simulink model "full_simulation_split_hil_new_connection"  (Simulink 7.9)
settings: Solver=ode1  StartTime=0  StopTime=10  FixedStep=Ts  RelTol=1e-8
values from neighbouring files (symbols this model uses):
  A_fx = 2e-2 * 0.4    (= 0.008)    [QR_DI_Init.m]    (also in quadro_cascade_disturbance_wo_wind.m)
  A_fy = A_fx    (= 0.008)    [QR_DI_Init.m]    (also in quadro_cascade_disturbance_wo_wind.m)
  A_fz = 2 * A_fx    (= 0.016)    [QR_DI_Init.m]    (also in quadro_cascade_disturbance_wo_wind.m)
  Bias_Phi = -0.0088    [QR_DI_Init.m]    (also in Reference_Calibration.m = mean(Phi))
  Bias_Theta = 0.022    [QR_DI_Init.m]    (also in Reference_Calibration.m = mean(Theta))
  command_on = 1    [QR_DI_Init.m]    (also in quadro_cascade_disturbance_wo_wind.m)
  cw_x = 1.05    [QR_DI_Init.m]    (also in quadro_cascade_disturbance_wo_wind.m)
  cw_y = cw_x    (= 1.05)    [QR_DI_Init.m]    (also in quadro_cascade_disturbance_wo_wind.m)
  cw_z = 1.05    [QR_DI_Init.m]    (also in quadro_cascade_disturbance_wo_wind.m)
  deltaTm = 0.2    [QR_DI_Init.m]    (also in quadro_cascade_disturbance_wo_wind.m)
  den_psi_ref = poly( ones(1,2) * -1 * T_psi_ref)    [QR_DI_Init.m]    (also in quadro_cascade_disturbance_wo_wind.m)
  den_x_ref = poly( ones(1,4) * -1 * T_x_ref)    [QR_DI_Init.m]    (also in quadro_cascade_disturbance_wo_wind.m)
  den_y_ref = poly( ones(1,4) * -1 * T_y_ref)    [QR_DI_Init.m]    (also in quadro_cascade_disturbance_wo_wind.m)
  den_z_ref = poly( ones(1,4) * -1 * T_z_ref)    [QR_DI_Init.m]    (also in quadro_cascade_disturbance_wo_wind.m)
  drot = 0.0117    [QR_DI_Init.m]    (also in quadro_cascade_disturbance_wo_wind.m = 0.2)
  dtran = 0.01    [QR_DI_Init.m]    (also in quadro_cascade_disturbance_wo_wind.m = 0.003)
  Fz_gain = 1 + 0.05*rand(1)    [QR_DI_Init.m]    (also in quadro_cascade_disturbance_wo_wind.m)
  Fz_lo = - 1.2 * m * g    (= -3.5316)    [QR_DI_Init.m]    (also in quadro_cascade_disturbance_wo_wind.m = -4.1202)
  Fz_up = 0    [QR_DI_Init.m]    (also in quadro_cascade_disturbance_wo_wind.m)
  g = 9.81    [QR_DI_Init.m]    (also in quadro_cascade_disturbance_wo_wind.m)
  Iq = [I_xx 0 0 ; 0 I_yy 0 ; 0 0 I_zz ]    [QR_DI_Init.m]    (also in quadro_cascade_disturbance_wo_wind.m = [0.0605 0 0; 0 0.0605 0; 0 0 0.018])
  K_err = old(:,2:end)    [QR_DI_Init.m]    (also in quadro_cascade_disturbance_wo_wind.m)
  K_Mot_Force = 0.3512    [QR_DI_Init.m]    (also in quadro_cascade_disturbance_wo_wind.m)
  K_Mot_Torque = 0.013    [QR_DI_Init.m]    (also in quadro_cascade_disturbance_wo_wind.m = 0.0013)
  l = 0.25    [QR_DI_Init.m]    (also in quadro_cascade_disturbance_wo_wind.m = 0.2775)
  m = 0.30    (= 0.3)    [QR_DI_Init.m]    (also in quadro_cascade_disturbance_wo_wind.m)
  m_real = m * ( 1 + 0.05*rand(1))    [QR_DI_Init.m]    (also in quadro_cascade_disturbance_wo_wind.m)
  Mm = 0.0    (= 0)    [QR_DI_Init.m]    (also in quadro_cascade_disturbance_wo_wind.m = 0.5)
  Mx_lo = - Mx_up    (= -0.2)    [QR_DI_Init.m]    (also in quadro_cascade_disturbance_wo_wind.m)
  Mx_up = 0.20    (= 0.2)    [QR_DI_Init.m]    (also in quadro_cascade_disturbance_wo_wind.m)
  My_lo = - My_up    (= -0.2)    [QR_DI_Init.m]    (also in quadro_cascade_disturbance_wo_wind.m)
  My_up = 0.20    (= 0.2)    [QR_DI_Init.m]    (also in quadro_cascade_disturbance_wo_wind.m)
  Mz_lo = - Mz_up    (= -0.02)    [QR_DI_Init.m]    (also in quadro_cascade_disturbance_wo_wind.m = -0.002)
  Mz_up = 0.02    [QR_DI_Init.m]    (also in quadro_cascade_disturbance_wo_wind.m = 0.002)
  phase_wind_z = 0    [QR_DI_Init.m]    (also in quadro_cascade_disturbance_wo_wind.m)
  psi_p_lim = 10*pi/180    (= 0.174532925199)    [QR_DI_Init.m]    (also in quadro_cascade_disturbance_wo_wind.m = 5)
  PWM_MAX = 200    [QR_DI_Init.m]    (also in quadro_cascade_disturbance_wo_wind.m)
  rho_air = 1.2041    [QR_DI_Init.m]    (also in quadro_cascade_disturbance_wo_wind.m)
  sample_time_noise_psi = 0.1    [QR_DI_Init.m]
  sample_time_noise_x = 0.2    [QR_DI_Init.m]
  sample_time_noise_y = 0.2    [QR_DI_Init.m]
  sample_time_noise_z = 0.1    [QR_DI_Init.m]
  seed_psi = seedvector(7)    [QR_DI_Init.m]
  seed_x = seedvector(1)    [QR_DI_Init.m]    (also in quadro_cascade_disturbance_wo_wind.m)
  seed_xp = seedvector(4)    [QR_DI_Init.m]    (also in quadro_cascade_disturbance_wo_wind.m)
  seed_y = seedvector(2)    [QR_DI_Init.m]    (also in quadro_cascade_disturbance_wo_wind.m)
  seed_yp = seedvector(5)    [QR_DI_Init.m]    (also in quadro_cascade_disturbance_wo_wind.m)
  seed_z = seedvector(3)    [QR_DI_Init.m]    (also in quadro_cascade_disturbance_wo_wind.m)
  seed_zp = seedvector(6)    [QR_DI_Init.m]    (also in quadro_cascade_disturbance_wo_wind.m)
  std_dev_psi = 1 * pi/180 * Noise_on    (= 0)    [QR_DI_Init.m]
  std_dev_x = 1e-1 * Noise_on    (= 0)    [QR_DI_Init.m]
  std_dev_xp = 0.03 * Noise_on    (= 0)    [QR_DI_Init.m]
  std_dev_y = 1e-1 * Noise_on    (= 0)    [QR_DI_Init.m]
  std_dev_yp = 0.03 * Noise_on    (= 0)    [QR_DI_Init.m]
  std_dev_z = 0.03 * Noise_on    (= 0)    [QR_DI_Init.m]
  std_dev_zp = 0.03 * Noise_on    (= 0)    [QR_DI_Init.m]
  T_refalt = 0.01    [QR_DI_Init.m]    (also in quadro_cascade_disturbance_wo_wind.m)
  T_wind_z = 24    [QR_DI_Init.m]    (also in quadro_cascade_disturbance_wo_wind.m)
  Tm = 10    [QR_DI_Init.m]    (also in quadro_cascade_disturbance_wo_wind.m)
  Ts = 1e-2    (= 0.01)    [QR_DI_Init.m]    (also in quadro_cascade_disturbance_wo_wind.m)
  v_wind_max_z = 2    [QR_DI_Init.m]    (also in quadro_cascade_disturbance_wo_wind.m)
  wind_on = 0    [QR_DI_Init.m]    (also in quadro_cascade_disturbance_wo_wind.m)
  x_p_lim = 1.5    [QR_DI_Init.m]    (also in quadro_cascade_disturbance_wo_wind.m = 5)
  y_p_lim = 1.5    [QR_DI_Init.m]    (also in quadro_cascade_disturbance_wo_wind.m = 5)
  z_p_lim = 1    [QR_DI_Init.m]    (also in quadro_cascade_disturbance_wo_wind.m = 1.5)
undefined symbols (not defined in the file or in its folder): T_wind_fine, v_wind_x_fine, v_wind_y_fine
libraries: simulink x5, dspsigops x4, Ports x4, aerolibtransform2 x3, dspmtrx3 x1, aerolibutil x1
(part 3 of 6)

== matlab function Error Dynamic/coordinate transformation1/Embedded MATLAB Function ==
  data: xwhole_ext input double size=[14 1]; xi output double size=14; m input double; I input double size=[3 3]; dtran input double; drot input double
% S.H. 26.03.2013
% new correct coordinate transformation

function xi  = fcn(xwhole_ext, m, I, dtran, drot)
% This block supports the Embedded MATLAB subset.
% See the help menu for details. 
x = xwhole_ext(1);
y = xwhole_ext(2);
z = xwhole_ext(3);
dx = xwhole_ext(4);
dy = xwhole_ext(5);
dz = xwhole_ext(6);

% phi = xwhole_ext(7);
% theta = xwhole_ext(8);
% psi = xwhole_ext(9);
% p = xwhole_ext(10);
% q = xwhole_ext(11);
% r = xwhole_ext(12);
% 
% xi1 = xwhole_ext(13) +eps;
% dxi1 = xwhole_ext(14) +eps;

% S.H. 26.03.2013 --> in order to match "controller_design_steps.m"
phi_angle = xwhole_ext(7);
theta_angle = xwhole_ext(8);
psi_angle = xwhole_ext(9);
p = xwhole_ext(10);
q = xwhole_ext(11);
r = xwhole_ext(12);

Sym_zeta    = xwhole_ext(13) +eps;
Sym_zeta_p  = xwhole_ext(14) +eps;


%g = -9.81;
g = 9.81;   % S.H. 26.03.2013


Ixx = I(1,1);
Ixy = I(1,2);
Ixz = I(1,3);
Iyy = I(2,2);
Iyz = I(2,3);
Izz = I(3,3);

output = zeros(14,1); 

% output(1,1) = x;
% output(2,1) = dx;
% output(3,1) = -dtran*dx+xi1/m*(sin(psi)*sin(phi)+cos(psi)*cos(phi)*sin(theta));
% output(4,1) = -dtran*(-dtran*dx+xi1/m*(sin(psi)*sin(phi)+cos(psi)*cos(phi)*sin(theta)))+xi1/m*(sin(psi)*cos(phi)-cos(psi)*sin(phi)*sin(theta))*(p+sin(phi)*tan(theta)*q+cos(phi)*tan(theta)*r)+xi1/m*cos(psi)*cos(phi)*cos(theta)*(cos(phi)*q-sin(phi)*r)+xi1/m*(-cos(phi)*sin(psi)*sin(theta)+cos(psi)*sin(phi))*(sin(phi)/cos(theta)*q+cos(phi)/cos(theta)*r)+1/m*(sin(psi)*sin(phi)+cos(psi)*cos(phi)*sin(theta))*dxi1;
% output(5,1) = dtran^2*(-dtran*dx+xi1/m*(sin(psi)*sin(phi)+cos(psi)*cos(phi)*sin(theta)))+(-dtran*xi1/m*(sin(psi)*cos(phi)-cos(psi)*sin(phi)*sin(theta))+xi1/m*(-sin(psi)*sin(phi)-cos(psi)*cos(phi)*sin(theta))*(p+sin(phi)*tan(theta)*q+cos(phi)*tan(theta)*r)+xi1/m*(sin(psi)*cos(phi)-cos(psi)*sin(phi)*sin(theta))*(cos(phi)*tan(theta)*q-sin(phi)*tan(theta)*r)-xi1/m*cos(psi)*sin(phi)*cos(theta)*(cos(phi)*q-sin(phi)*r)+xi1/m*cos(psi)*cos(phi)*cos(theta)*(-sin(phi)*q-cos(phi)*r)+xi1/m*(sin(phi)*sin(psi)*sin(theta)+cos(psi)*cos(phi))*(sin(phi)/cos(theta)*q+cos(phi)/cos(theta)*r)+xi1/m*(-cos(phi)*sin(psi)*sin(theta)+cos(psi)*sin(phi))*(cos(phi)/cos(theta)*q-sin(phi)/cos(theta)*r)+1/m*(sin(psi)*cos(phi)-cos(psi)*sin(phi)*sin(theta))*dxi1)*(p+sin(phi)*tan(theta)*q+cos(phi)*tan(theta)*r)+(-dtran*xi1/m*cos(psi)*cos(phi)*cos(theta)-xi1/m*cos(psi)*sin(phi)*cos(theta)*(p+sin(phi)*tan(theta)*q+cos(phi)*tan(theta)*r)+xi1/m*(sin(psi)*cos(phi)-cos(psi)*sin(phi)*sin(theta))*(sin(phi)*(1+tan(theta)^2)*q+cos(phi)*(1+tan(theta)^2)*r)-xi1/m*cos(psi)*cos(phi)*sin(theta)*(cos(phi)*q-sin(phi)*r)-xi1/m*cos(phi)*sin(psi)*cos(theta)*(sin(phi)/cos(theta)*q+cos(phi)/cos(theta)*r)+xi1/m*(-cos(phi)*sin(psi)*sin(theta)+cos(psi)*sin(phi))*(sin(phi)/cos(theta)^2*q*sin(theta)+cos(phi)/cos(theta)^2*r*sin(theta))+1/m*cos(psi)*cos(phi)*cos(theta)*dxi1)*(cos(phi)*q-sin(phi)*r)+(-dtran*xi1/m*(-cos(phi)*sin(psi)*sin(theta)+cos(psi)*sin(phi))+xi1/m*(sin(phi)*sin(psi)*sin(theta)+cos(psi)*cos(phi))*(p+sin(phi)*tan(theta)*q+cos(phi)*tan(theta)*r)-xi1/m*sin(psi)*cos(phi)*cos(theta)*(cos(phi)*q-sin(phi)*r)+xi1/m*(-sin(psi)*sin(phi)-cos(psi)*cos(phi)*sin(theta))*(sin(phi)/cos(theta)*q+cos(phi)/cos(theta)*r)+1/m*(-cos(phi)*sin(psi)*sin(theta)+cos(psi)*sin(phi))*dxi1)*(sin(phi)/cos(theta)*q+cos(phi)/cos(theta)*r)+xi1/m*(sin(psi)*cos(phi)-cos(psi)*sin(phi)*sin(theta))*(-drot*p-1/Ixx*(q*Izz*r-r*Iyy*q))+(xi1/m*(sin(psi)*cos(phi)-cos(psi)*sin(phi)*sin(theta))*sin(phi)*tan(theta)+xi1/m*cos(psi)*cos(phi)^2*cos(theta)+xi1/m*(-cos(phi)*sin(psi)*sin(theta)+cos(psi)*sin(phi))*sin(phi)/cos(theta))*(-drot*q-1/Iyy*(r*Ixx*p-p*Izz*r))+(xi1/m*(sin(psi)*cos(phi)-cos(psi)*sin(phi)*sin(theta))*cos(phi)*tan(theta)-xi1/m*cos(psi)*cos(phi)*cos(theta)*sin(phi)+xi1/m*(-cos(phi)*sin(psi)*sin(theta)+cos(psi)*sin(phi))*cos(phi)/cos(theta))*(-drot*r-1/Izz*(p*Iyy*q-q*Ixx*p))+(-dtran/m*(sin(psi)*sin(phi)+cos(psi)*cos(phi)*sin(theta))+1/m*(sin(psi)*cos(phi)-cos(psi)*sin(phi)*sin(theta))*(p+sin(phi)*tan(theta)*q+cos(phi)*tan(theta)*r)+1/m*cos(psi)*cos(phi)*cos(theta)*(cos(phi)*q-sin(phi)*r)+1/m*(-cos(phi)*sin(psi)*sin(theta)+cos(psi)*sin(phi))*(sin(phi)/cos(theta)*q+cos(phi)/cos(theta)*r))*dxi1;
% output(6,1) = y;
% output(7,1) = dy;
% output(8,1) = -dtran*dy+xi1/m*(cos(phi)*sin(psi)*sin(theta)-cos(psi)*sin(phi));
% output(9,1) = -dtran*(-dtran*dy+xi1/m*(cos(phi)*sin(psi)*sin(theta)-cos(psi)*sin(phi)))+xi1/m*(-sin(phi)*sin(psi)*sin(theta)-cos(psi)*cos(phi))*(p+sin(phi)*tan(theta)*q+cos(phi)*tan(theta)*r)+xi1/m*sin(psi)*cos(phi)*cos(theta)*(cos(phi)*q-sin(phi)*r)+xi1/m*(sin(psi)*sin(phi)+cos(psi)*cos(phi)*sin(theta))*(sin(phi)/cos(theta)*q+cos(phi)/cos(theta)*r)+1/m*(cos(phi)*sin(psi)*sin(theta)-cos(psi)*sin(phi))*dxi1;
% output(10,1) = dtran^2*(-dtran*dy+xi1/m*(cos(phi)*sin(psi)*sin(theta)-cos(psi)*sin(phi)))+(-dtran*xi1/m*(-sin(phi)*sin(psi)*sin(theta)-cos(psi)*cos(phi))+xi1/m*(-cos(phi)*sin(psi)*sin(theta)+cos(psi)*sin(phi))*(p+sin(phi)*tan(theta)*q+cos(phi)*tan(theta)*r)+xi1/m*(-sin(phi)*sin(psi)*sin(theta)-cos(psi)*cos(phi))*(cos(phi)*tan(theta)*q-sin(phi)*tan(theta)*r)-xi1/m*sin(psi)*sin(phi)*cos(theta)*(cos(phi)*q-sin(phi)*r)+xi1/m*sin(psi)*cos(phi)*cos(theta)*(-sin(phi)*q-cos(phi)*r)+xi1/m*(sin(psi)*cos(phi)-cos(psi)*sin(phi)*sin(theta))*(sin(phi)/cos(theta)*q+cos(phi)/cos(theta)*r)+xi1/m*(sin(psi)*sin(phi)+cos(psi)*cos(phi)*sin(theta))*(cos(phi)/cos(theta)*q-sin(phi)/cos(theta)*r)+1/m*(-sin(phi)*sin(psi)*sin(theta)-cos(psi)*cos(phi))*dxi1)*(p+sin(phi)*tan(theta)*q+cos(phi)*tan(theta)*r)+(-dtran*xi1/m*cos(phi)*sin(psi)*cos(theta)-xi1/m*sin(phi)*sin(psi)*cos(theta)*(p+sin(phi)*tan(theta)*q+cos(phi)*tan(theta)*r)+xi1/m*(-sin(phi)*sin(psi)*sin(theta)-cos(psi)*cos(phi))*(sin(phi)*(1+tan(theta)^2)*q+cos(phi)*(1+tan(theta)^2)*r)-xi1/m*sin(psi)*cos(phi)*sin(theta)*(cos(phi)*q-sin(phi)*r)+xi1/m*cos(psi)*cos(phi)*cos(theta)*(sin(phi)/cos(theta)*q+cos(phi)/cos(theta)*r)+xi1/m*(sin(psi)*sin(phi)+cos(psi)*cos(phi)*sin(theta))*(sin(phi)/cos(theta)^2*q*sin(theta)+cos(phi)/cos(theta)^2*r*sin(theta))+1/m*cos(phi)*sin(psi)*cos(theta)*dxi1)*(cos(phi)*q-sin(phi)*r)+(-dtran*xi1/m*(sin(psi)*sin(phi)+cos(psi)*cos(phi)*sin(theta))+xi1/m*(sin(psi)*cos(phi)-cos(psi)*sin(phi)*sin(theta))*(p+sin(phi)*tan(theta)*q+cos(phi)*tan(theta)*r)+xi1/m*cos(psi)*cos(phi)*cos(theta)*(cos(phi)*q-sin(phi)*r)+xi1/m*(-cos(phi)*sin(psi)*sin(theta)+cos(psi)*sin(phi))*(sin(phi)/cos(theta)*q+cos(phi)/cos(theta)*r)+1/m*(sin(psi)*sin(phi)+cos(psi)*cos(phi)*sin(theta))*dxi1)*(sin(phi)/cos(theta)*q+cos(phi)/cos(theta)*r)+xi1/m*(-sin(phi)*sin(psi)*sin(theta)-cos(psi)*cos(phi))*(-drot*p-1/Ixx*(q*Izz*r-r*Iyy*q))+(xi1/m*(-sin(phi)*sin(psi)*sin(theta)-cos(psi)*cos(phi))*sin(phi)*tan(theta)+xi1/m*sin(psi)*cos(phi)^2*cos(theta)+xi1/m*(sin(psi)*sin(phi)+cos(psi)*cos(phi)*sin(theta))*sin(phi)/cos(theta))*(-drot*q-1/Iyy*(r*Ixx*p-p*Izz*r))+(xi1/m*(-sin(phi)*sin(psi)*sin(theta)-cos(psi)*cos(phi))*cos(phi)*tan(theta)-xi1/m*sin(psi)*cos(phi)*cos(theta)*sin(phi)+xi1/m*(sin(psi)*sin(phi)+cos(psi)*cos(phi)*sin(theta))*cos(phi)/cos(theta))*(-drot*r-1/Izz*(p*Iyy*q-q*Ixx*p))+(-dtran/m*(cos(phi)*sin(psi)*sin(theta)-cos(psi)*sin(phi))+1/m*(-sin(phi)*sin(psi)*sin(theta)-cos(psi)*cos(phi))*(p+sin(phi)*tan(theta)*q+cos(phi)*tan(theta)*r)+1/m*sin(psi)*cos(phi)*cos(theta)*(cos(phi)*q-sin(phi)*r)+1/m*(sin(psi)*sin(phi)+cos(psi)*cos(phi)*sin(theta))*(sin(phi)/cos(theta)*q+cos(phi)/cos(theta)*r))*dxi1;
% output(11,1) = z;
% output(12,1) = dz;
% output(13,1) = -dtran*dz-m*g+xi1/m*cos(theta)*cos(phi);
% output(14,1) = -dtran*(-dtran*dz-m*g+xi1/m*cos(theta)*cos(phi))-xi1/m*cos(theta)*sin(phi)*(p+sin(phi)*tan(theta)*q+cos(phi)*tan(theta)*r)-xi1/m*sin(theta)*cos(phi)*(cos(phi)*q-sin(phi)*r)+1/m*cos(theta)*cos(phi)*dxi1 ;
% output(15,1) = dtran^2*(-dtran*dz-m*g+xi1/m*cos(theta)*cos(phi))+(dtran*xi1/m*cos(theta)*sin(phi)-xi1/m*cos(theta)*cos(phi)*(p+sin(phi)*tan(theta)*q+cos(phi)*tan(theta)*r)-xi1/m*cos(theta)*sin(phi)*(cos(phi)*tan(theta)*q-sin(phi)*tan(theta)*r)+xi1/m*sin(theta)*sin(phi)*(cos(phi)*q-sin(phi)*r)-xi1/m*sin(theta)*cos(phi)*(-sin(phi)*q-cos(phi)*r)-1/m*cos(theta)*sin(phi)*dxi1)*(p+sin(phi)*tan(theta)*q+cos(phi)*tan(theta)*r)+(dtran*xi1/m*sin(theta)*cos(phi)+xi1/m*sin(theta)*sin(phi)*(p+sin(phi)*tan(theta)*q+cos(phi)*tan(theta)*r)-xi1/m*cos(theta)*sin(phi)*(sin(phi)*(1+tan(theta)^2)*q+cos(phi)*(1+tan(theta)^2)*r)-xi1/m*cos(theta)*cos(phi)*(cos(phi)*q-sin(phi)*r)-1/m*sin(theta)*cos(phi)*dxi1)*(cos(phi)*q-sin(phi)*r)-xi1/m*cos(theta)*sin(phi)*(-drot*p-1/Ixx*(q*Izz*r-r*Iyy*q))+(-xi1/m*cos(theta)*sin(phi)^2*tan(theta)-xi1/m*sin(theta)*cos(phi)^2)*(-drot*q-1/Iyy*(r*Ixx*p-p*Izz*r))+(-xi1/m*cos(theta)*sin(phi)*cos(phi)*tan(theta)+xi1/m*sin(theta)*cos(phi)*sin(phi))*(-drot*r-1/Izz*(p*Iyy*q-q*Ixx*p))+(-dtran/m*cos(theta)*cos(phi)-1/m*cos(theta)*sin(phi)*(p+sin(phi)*tan(theta)*q+cos(phi)*tan(theta)*r)-1/m*sin(theta)*cos(phi)*(cos(phi)*q-sin(phi)*r))*dxi1; 
% output(16,1) =  psi;
% output(17,1) = sin(phi)/cos(theta)*q+cos(phi)/cos(theta)*r;
% output(18,1) = (cos(phi)/cos(theta)*q-sin(phi)/cos(theta)*r)*(p+sin(phi)*tan(theta)*q+cos(phi)*tan(theta)*r)+(sin(phi)/cos(theta)^2*q*sin(theta)+cos(phi)/cos(theta)^2*r*sin(theta))*(cos(phi)*q-sin(phi)*r)+sin(phi)/cos(theta)*(-drot*q-1/Iyy*(r*Ixx*p-p*Izz*r))+cos(phi)/cos(theta)*(-drot*r-1/Izz*(p*Iyy*q-q*Ixx*p));

% Old
% output(1,1) = x;
% output(2,1) = dx;
% output(3,1) = -dtran*dx+xi1/m*(sin(psi)*sin(phi)+cos(psi)*cos(phi)*sin(theta));
% output(4,1) = -dtran*(-dtran*dx+xi1/m*(sin(psi)*sin(phi)+cos(psi)*cos(phi)*sin(theta)))+xi1/m*(sin(psi)*cos(phi)-cos(psi)*sin(phi)*sin(theta))*(p+sin(phi)*tan(theta)*q+cos(phi)*tan(theta)*r)+xi1/m*cos(psi)*cos(phi)*cos(theta)*(cos(phi)*q-sin(phi)*r)+xi1/m*(-cos(phi)*sin(psi)*sin(theta)+cos(psi)*sin(phi))*(sin(phi)/cos(theta)*q+cos(phi)/cos(theta)*r)+1/m*(sin(psi)*sin(phi)+cos(psi)*cos(phi)*sin(theta))*dxi1;
% output(5,1) = y;
% output(6,1) = dy;
% output(7,1) = -dtran*dy+xi1/m*(cos(phi)*sin(psi)*sin(theta)-cos(psi)*sin(phi));
% output(8,1) = -dtran*(-dtran*dy+xi1/m*(cos(phi)*sin(psi)*sin(theta)-cos(psi)*sin(phi)))+xi1/m*(-sin(phi)*sin(psi)*sin(theta)-cos(psi)*cos(phi))*(p+sin(phi)*tan(theta)*q+cos(phi)*tan(theta)*r)+xi1/m*sin(psi)*cos(phi)*cos(theta)*(cos(phi)*q-sin(phi)*r)+xi1/m*(sin(psi)*sin(phi)+cos(psi)*cos(phi)*sin(theta))*(sin(phi)/cos(theta)*q+cos(phi)/cos(theta)*r)+1/m*(cos(phi)*sin(psi)*sin(theta)-cos(psi)*sin(phi))*dxi1;
% output(9,1) = z;
% output(10,1) = dz;
% output(11,1) = -dtran*dz-m*g+xi1/m*cos(theta)*cos(phi);
% output(12,1) = -dtran*(-dtran*dz-m*g+xi1/m*cos(theta)*cos(phi))-xi1/m*cos(theta)*sin(phi)*(p+sin(phi)*tan(theta)*q+cos(phi)*tan(theta)*r)-xi1/m*sin(theta)*cos(phi)*(cos(phi)*q-sin(phi)*r)+1/m*cos(theta)*cos(phi)*dxi1 ;
% output(13,1) =  psi;
% output(14,1) = sin(phi)/cos(theta)*q+cos(phi)/cos(theta)*r;

% S.H. 26.03.2013
output(1,1) = x;
output(2,1) = dx;
output(3,1) =  (Sym_zeta*(sin(phi_angle)*sin(psi_angle) + cos(phi_angle)*cos(psi_angle)*sin(theta_angle)))/m - (dtran*dx)/m;
output(4,1) = (dtran*((dtran*dx)/m - (Sym_zeta*(sin(phi_angle)*sin(psi_angle) + cos(phi_angle)*cos(psi_angle)*sin(theta_angle)))/m))/m + (Sym_zeta_p*(sin(phi_angle)*sin(psi_angle) + cos(phi_angle)*cos(psi_angle)*sin(theta_angle)))/m + (Sym_zeta*((r*cos(phi_angle))/cos(theta_angle) + (q*sin(phi_angle))/cos(theta_angle))*(cos(psi_angle)*sin(phi_angle) - cos(phi_angle)*sin(psi_angle)*sin(theta_angle)))/m + (Sym_zeta*(cos(phi_angle)*sin(psi_angle) - cos(psi_angle)*sin(phi_angle)*sin(theta_angle))*(p + r*cos(phi_angle)*tan(theta_angle) + q*sin(phi_angle)*tan(theta_angle)))/m + (Sym_zeta*cos(phi_angle)*cos(psi_angle)*cos(theta_angle)*(q*cos(phi_angle) - r*sin(phi_angle)))/m;
output(5,1) = y;
output(6,1) = dy;
output(7,1) =  - (dtran*dy)/m - (Sym_zeta*(cos(psi_angle)*sin(phi_angle) - cos(phi_angle)*sin(psi_angle)*sin(theta_angle)))/m;
output(8,1) = (dtran*((dtran*dy)/m + (Sym_zeta*(cos(psi_angle)*sin(phi_angle) - cos(phi_angle)*sin(psi_angle)*sin(theta_angle)))/m))/m - (Sym_zeta_p*(cos(psi_angle)*sin(phi_angle) - cos(phi_angle)*sin(psi_angle)*sin(theta_angle)))/m + (Sym_zeta*((r*cos(phi_angle))/cos(theta_angle) + (q*sin(phi_angle))/cos(theta_angle))*(sin(phi_angle)*sin(psi_angle) + cos(phi_angle)*cos(psi_angle)*sin(theta_angle)))/m - (Sym_zeta*(cos(phi_angle)*cos(psi_angle) + sin(phi_angle)*sin(psi_angle)*sin(theta_angle))*(p + r*cos(phi_angle)*tan(theta_angle) + q*sin(phi_angle)*tan(theta_angle)))/m + (Sym_zeta*cos(phi_angle)*cos(theta_angle)*sin(psi_angle)*(q*cos(phi_angle) - r*sin(phi_angle)))/m;
output(9,1) = z;
output(10,1) = dz;
output(11,1) = g - (dtran*dz)/m + (Sym_zeta*cos(phi_angle)*cos(theta_angle))/m;
output(12,1) = (Sym_zeta_p*cos(phi_angle)*cos(theta_angle))/m - (dtran*(g - (dtran*dz)/m + (Sym_zeta*cos(phi_angle)*cos(theta_angle))/m))/m - (Sym_zeta*cos(theta_angle)*sin(phi_angle)*(p + r*cos(phi_angle)*tan(theta_angle) + q*sin(phi_angle)*tan(theta_angle)))/m - (Sym_zeta*cos(phi_angle)*sin(theta_angle)*(q*cos(phi_angle) - r*sin(phi_angle)))/m;
output(13,1) =  psi_angle;
output(14,1) =  (r*cos(phi_angle))/cos(theta_angle) + (q*sin(phi_angle))/cos(theta_angle); 

xi = output;


%% Old

% % % function xi  = fcn(xwhole_ext, m, I, dtran, drot)
% % % % This block supports the Embedded MATLAB subset.
% % % % See the help menu for details. 
% % % x = xwhole_ext(1);
% % % y = xwhole_ext(2);
% % % z = xwhole_ext(3);
% % % dx = xwhole_ext(4);
% % % dy = xwhole_ext(5);
% % % dz = xwhole_ext(6);
% % % 
% % % phi = xwhole_ext(7);
% % % theta = xwhole_ext(8);
% % % psi = xwhole_ext(9);
% % % p = xwhole_ext(10);
% % % q = xwhole_ext(11);
% % % r = xwhole_ext(12);
% % % 
% % % xi1 = xwhole_ext(13) +eps;
% % % dxi1 = xwhole_ext(14) +eps;
% % % 
% % % 
% % % 
% % % 
% % % g = -9.81;
% % % 
% % % 
% % % Ixx = I(1,1);
% % % Ixy = I(1,2);
% % % Ixz = I(1,3);
% % % Iyy = I(2,2);
% % % Iyz = I(2,3);
% % % Izz = I(3,3);
% % % 
% % % output = zeros(14,1); 
% % % 
% % % % output(1,1) = x;
% % % % output(2,1) = dx;
% % % % output(3,1) = -dtran*dx+xi1/m*(sin(psi)*sin(phi)+cos(psi)*cos(phi)*sin(theta));
% % % % output(4,1) = -dtran*(-dtran*dx+xi1/m*(sin(psi)*sin(phi)+cos(psi)*cos(phi)*sin(theta)))+xi1/m*(sin(psi)*cos(phi)-cos(psi)*sin(phi)*sin(theta))*(p+sin(phi)*tan(theta)*q+cos(phi)*tan(theta)*r)+xi1/m*cos(psi)*cos(phi)*cos(theta)*(cos(phi)*q-sin(phi)*r)+xi1/m*(-cos(phi)*sin(psi)*sin(theta)+cos(psi)*sin(phi))*(sin(phi)/cos(theta)*q+cos(phi)/cos(theta)*r)+1/m*(sin(psi)*sin(phi)+cos(psi)*cos(phi)*sin(theta))*dxi1;
% % % % output(5,1) = dtran^2*(-dtran*dx+xi1/m*(sin(psi)*sin(phi)+cos(psi)*cos(phi)*sin(theta)))+(-dtran*xi1/m*(sin(psi)*cos(phi)-cos(psi)*sin(phi)*sin(theta))+xi1/m*(-sin(psi)*sin(phi)-cos(psi)*cos(phi)*sin(theta))*(p+sin(phi)*tan(theta)*q+cos(phi)*tan(theta)*r)+xi1/m*(sin(psi)*cos(phi)-cos(psi)*sin(phi)*sin(theta))*(cos(phi)*tan(theta)*q-sin(phi)*tan(theta)*r)-xi1/m*cos(psi)*sin(phi)*cos(theta)*(cos(phi)*q-sin(phi)*r)+xi1/m*cos(psi)*cos(phi)*cos(theta)*(-sin(phi)*q-cos(phi)*r)+xi1/m*(sin(phi)*sin(psi)*sin(theta)+cos(psi)*cos(phi))*(sin(phi)/cos(theta)*q+cos(phi)/cos(theta)*r)+xi1/m*(-cos(phi)*sin(psi)*sin(theta)+cos(psi)*sin(phi))*(cos(phi)/cos(theta)*q-sin(phi)/cos(theta)*r)+1/m*(sin(psi)*cos(phi)-cos(psi)*sin(phi)*sin(theta))*dxi1)*(p+sin(phi)*tan(theta)*q+cos(phi)*tan(theta)*r)+(-dtran*xi1/m*cos(psi)*cos(phi)*cos(theta)-xi1/m*cos(psi)*sin(phi)*cos(theta)*(p+sin(phi)*tan(theta)*q+cos(phi)*tan(theta)*r)+xi1/m*(sin(psi)*cos(phi)-cos(psi)*sin(phi)*sin(theta))*(sin(phi)*(1+tan(theta)^2)*q+cos(phi)*(1+tan(theta)^2)*r)-xi1/m*cos(psi)*cos(phi)*sin(theta)*(cos(phi)*q-sin(phi)*r)-xi1/m*cos(phi)*sin(psi)*cos(theta)*(sin(phi)/cos(theta)*q+cos(phi)/cos(theta)*r)+xi1/m*(-cos(phi)*sin(psi)*sin(theta)+cos(psi)*sin(phi))*(sin(phi)/cos(theta)^2*q*sin(theta)+cos(phi)/cos(theta)^2*r*sin(theta))+1/m*cos(psi)*cos(phi)*cos(theta)*dxi1)*(cos(phi)*q-sin(phi)*r)+(-dtran*xi1/m*(-cos(phi)*sin(psi)*sin(theta)+cos(psi)*sin(phi))+xi1/m*(sin(phi)*sin(psi)*sin(theta)+cos(psi)*cos(phi))*(p+sin(phi)*tan(theta)*q+cos(phi)*tan(theta)*r)-xi1/m*sin(psi)*cos(phi)*cos(theta)*(cos(phi)*q-sin(phi)*r)+xi1/m*(-sin(psi)*sin(phi)-cos(psi)*cos(phi)*sin(theta))*(sin(phi)/cos(theta)*q+cos(phi)/cos(theta)*r)+1/m*(-cos(phi)*sin(psi)*sin(theta)+cos(psi)*sin(phi))*dxi1)*(sin(phi)/cos(theta)*q+cos(phi)/cos(theta)*r)+xi1/m*(sin(psi)*cos(phi)-cos(psi)*sin(phi)*sin(theta))*(-drot*p-1/Ixx*(q*Izz*r-r*Iyy*q))+(xi1/m*(sin(psi)*cos(phi)-cos(psi)*sin(phi)*sin(theta))*sin(phi)*tan(theta)+xi1/m*cos(psi)*cos(phi)^2*cos(theta)+xi1/m*(-cos(phi)*sin(psi)*sin(theta)+cos(psi)*sin(phi))*sin(phi)/cos(theta))*(-drot*q-1/Iyy*(r*Ixx*p-p*Izz*r))+(xi1/m*(sin(psi)*cos(phi)-cos(psi)*sin(phi)*sin(theta))*cos(phi)*tan(theta)-xi1/m*cos(psi)*cos(phi)*cos(theta)*sin(phi)+xi1/m*(-cos(phi)*sin(psi)*sin(theta)+cos(psi)*sin(phi))*cos(phi)/cos(theta))*(-drot*r-1/Izz*(p*Iyy*q-q*Ixx*p))+(-dtran/m*(sin(psi)*sin(phi)+cos(psi)*cos(phi)*sin(theta))+1/m*(sin(psi)*cos(phi)-cos(psi)*sin(phi)*sin(theta))*(p+sin(phi)*tan(theta)*q+cos(phi)*tan(theta)*r)+1/m*cos(psi)*cos(phi)*cos(theta)*(cos(phi)*q-sin(phi)*r)+1/m*(-cos(phi)*sin(psi)*sin(theta)+cos(psi)*sin(phi))*(sin(phi)/cos(theta)*q+cos(phi)/cos(theta)*r))*dxi1;
% % % % output(6,1) = y;
% % % % output(7,1) = dy;
% % % % output(8,1) = -dtran*dy+xi1/m*(cos(phi)*sin(psi)*sin(theta)-cos(psi)*sin(phi));
% % % % output(9,1) = -dtran*(-dtran*dy+xi1/m*(cos(phi)*sin(psi)*sin(theta)-cos(psi)*sin(phi)))+xi1/m*(-sin(phi)*sin(psi)*sin(theta)-cos(psi)*cos(phi))*(p+sin(phi)*tan(theta)*q+cos(phi)*tan(theta)*r)+xi1/m*sin(psi)*cos(phi)*cos(theta)*(cos(phi)*q-sin(phi)*r)+xi1/m*(sin(psi)*sin(phi)+cos(psi)*cos(phi)*sin(theta))*(sin(phi)/cos(theta)*q+cos(phi)/cos(theta)*r)+1/m*(cos(phi)*sin(psi)*sin(theta)-cos(psi)*sin(phi))*dxi1;
% % % % output(10,1) = dtran^2*(-dtran*dy+xi1/m*(cos(phi)*sin(psi)*sin(theta)-cos(psi)*sin(phi)))+(-dtran*xi1/m*(-sin(phi)*sin(psi)*sin(theta)-cos(psi)*cos(phi))+xi1/m*(-cos(phi)*sin(psi)*sin(theta)+cos(psi)*sin(phi))*(p+sin(phi)*tan(theta)*q+cos(phi)*tan(theta)*r)+xi1/m*(-sin(phi)*sin(psi)*sin(theta)-cos(psi)*cos(phi))*(cos(phi)*tan(theta)*q-sin(phi)*tan(theta)*r)-xi1/m*sin(psi)*sin(phi)*cos(theta)*(cos(phi)*q-sin(phi)*r)+xi1/m*sin(psi)*cos(phi)*cos(theta)*(-sin(phi)*q-cos(phi)*r)+xi1/m*(sin(psi)*cos(phi)-cos(psi)*sin(phi)*sin(theta))*(sin(phi)/cos(theta)*q+cos(phi)/cos(theta)*r)+xi1/m*(sin(psi)*sin(phi)+cos(psi)*cos(phi)*sin(theta))*(cos(phi)/cos(theta)*q-sin(phi)/cos(theta)*r)+1/m*(-sin(phi)*sin(psi)*sin(theta)-cos(psi)*cos(phi))*dxi1)*(p+sin(phi)*tan(theta)*q+cos(phi)*tan(theta)*r)+(-dtran*xi1/m*cos(phi)*sin(psi)*cos(theta)-xi1/m*sin(phi)*sin(psi)*cos(theta)*(p+sin(phi)*tan(theta)*q+cos(phi)*tan(theta)*r)+xi1/m*(-sin(phi)*sin(psi)*sin(theta)-cos(psi)*cos(phi))*(sin(phi)*(1+tan(theta)^2)*q+cos(phi)*(1+tan(theta)^2)*r)-xi1/m*sin(psi)*cos(phi)*sin(theta)*(cos(phi)*q-sin(phi)*r)+xi1/m*cos(psi)*cos(phi)*cos(theta)*(sin(phi)/cos(theta)*q+cos(phi)/cos(theta)*r)+xi1/m*(sin(psi)*sin(phi)+cos(psi)*cos(phi)*sin(theta))*(sin(phi)/cos(theta)^2*q*sin(theta)+cos(phi)/cos(theta)^2*r*sin(theta))+1/m*cos(phi)*sin(psi)*cos(theta)*dxi1)*(cos(phi)*q-sin(phi)*r)+(-dtran*xi1/m*(sin(psi)*sin(phi)+cos(psi)*cos(phi)*sin(theta))+xi1/m*(sin(psi)*cos(phi)-cos(psi)*sin(phi)*sin(theta))*(p+sin(phi)*tan(theta)*q+cos(phi)*tan(theta)*r)+xi1/m*cos(psi)*cos(phi)*cos(theta)*(cos(phi)*q-sin(phi)*r)+xi1/m*(-cos(phi)*sin(psi)*sin(theta)+cos(psi)*sin(phi))*(sin(phi)/cos(theta)*q+cos(phi)/cos(theta)*r)+1/m*(sin(psi)*sin(phi)+cos(psi)*cos(phi)*sin(theta))*dxi1)*(sin(phi)/cos(theta)*q+cos(phi)/cos(theta)*r)+xi1/m*(-sin(phi)*sin(psi)*sin(theta)-cos(psi)*cos(phi))*(-drot*p-1/Ixx*(q*Izz*r-r*Iyy*q))+(xi1/m*(-sin(phi)*sin(psi)*sin(theta)-cos(psi)*cos(phi))*sin(phi)*tan(theta)+xi1/m*sin(psi)*cos(phi)^2*cos(theta)+xi1/m*(sin(psi)*sin(phi)+cos(psi)*cos(phi)*sin(theta))*sin(phi)/cos(theta))*(-drot*q-1/Iyy*(r*Ixx*p-p*Izz*r))+(xi1/m*(-sin(phi)*sin(psi)*sin(theta)-cos(psi)*cos(phi))*cos(phi)*tan(theta)-xi1/m*sin(psi)*cos(phi)*cos(theta)*sin(phi)+xi1/m*(sin(psi)*sin(phi)+cos(psi)*cos(phi)*sin(theta))*cos(phi)/cos(theta))*(-drot*r-1/Izz*(p*Iyy*q-q*Ixx*p))+(-dtran/m*(cos(phi)*sin(psi)*sin(theta)-cos(psi)*sin(phi))+1/m*(-sin(phi)*sin(psi)*sin(theta)-cos(psi)*cos(phi))*(p+sin(phi)*tan(theta)*q+cos(phi)*tan(theta)*r)+1/m*sin(psi)*cos(phi)*cos(theta)*(cos(phi)*q-sin(phi)*r)+1/m*(sin(psi)*sin(phi)+cos(psi)*cos(phi)*sin(theta))*(sin(phi)/cos(theta)*q+cos(phi)/cos(theta)*r))*dxi1;
% % % % output(11,1) = z;
% % % % output(12,1) = dz;
% % % % output(13,1) = -dtran*dz-m*g+xi1/m*cos(theta)*cos(phi);
% % % % output(14,1) = -dtran*(-dtran*dz-m*g+xi1/m*cos(theta)*cos(phi))-xi1/m*cos(theta)*sin(phi)*(p+sin(phi)*tan(theta)*q+cos(phi)*tan(theta)*r)-xi1/m*sin(theta)*cos(phi)*(cos(phi)*q-sin(phi)*r)+1/m*cos(theta)*cos(phi)*dxi1 ;
% % % % output(15,1) = dtran^2*(-dtran*dz-m*g+xi1/m*cos(theta)*cos(phi))+(dtran*xi1/m*cos(theta)*sin(phi)-xi1/m*cos(theta)*cos(phi)*(p+sin(phi)*tan(theta)*q+cos(phi)*tan(theta)*r)-xi1/m*cos(theta)*sin(phi)*(cos(phi)*tan(theta)*q-sin(phi)*tan(theta)*r)+xi1/m*sin(theta)*sin(phi)*(cos(phi)*q-sin(phi)*r)-xi1/m*sin(theta)*cos(phi)*(-sin(phi)*q-cos(phi)*r)-1/m*cos(theta)*sin(phi)*dxi1)*(p+sin(phi)*tan(theta)*q+cos(phi)*tan(theta)*r)+(dtran*xi1/m*sin(theta)*cos(phi)+xi1/m*sin(theta)*sin(phi)*(p+sin(phi)*tan(theta)*q+cos(phi)*tan(theta)*r)-xi1/m*cos(theta)*sin(phi)*(sin(phi)*(1+tan(theta)^2)*q+cos(phi)*(1+tan(theta)^2)*r)-xi1/m*cos(theta)*cos(phi)*(cos(phi)*q-sin(phi)*r)-1/m*sin(theta)*cos(phi)*dxi1)*(cos(phi)*q-sin(phi)*r)-xi1/m*cos(theta)*sin(phi)*(-drot*p-1/Ixx*(q*Izz*r-r*Iyy*q))+(-xi1/m*cos(theta)*sin(phi)^2*tan(theta)-xi1/m*sin(theta)*cos(phi)^2)*(-drot*q-1/Iyy*(r*Ixx*p-p*Izz*r))+(-xi1/m*cos(theta)*sin(phi)*cos(phi)*tan(theta)+xi1/m*sin(theta)*cos(phi)*sin(phi))*(-drot*r-1/Izz*(p*Iyy*q-q*Ixx*p))+(-dtran/m*cos(theta)*cos(phi)-1/m*cos(theta)*sin(phi)*(p+sin(phi)*tan(theta)*q+cos(phi)*tan(theta)*r)-1/m*sin(theta)*cos(phi)*(cos(phi)*q-sin(phi)*r))*dxi1; 
% % % % output(16,1) =  psi;
% % % % output(17,1) = sin(phi)/cos(theta)*q+cos(phi)/cos(theta)*r;
% % % % output(18,1) = (cos(phi)/cos(theta)*q-sin(phi)/cos(theta)*r)*(p+sin(phi)*tan(theta)*q+cos(phi)*tan(theta)*r)+(sin(phi)/cos(theta)^2*q*sin(theta)+cos(phi)/cos(theta)^2*r*sin(theta))*(cos(phi)*q-sin(phi)*r)+sin(phi)/cos(theta)*(-drot*q-1/Iyy*(r*Ixx*p-p*Izz*r))+cos(phi)/cos(theta)*(-drot*r-1/Izz*(p*Iyy*q-q*Ixx*p));
% % % output(1,1) = x;
% % % output(2,1) = dx;
% % % output(3,1) = -dtran*dx+xi1/m*(sin(psi)*sin(phi)+cos(psi)*cos(phi)*sin(theta));
% % % output(4,1) = -dtran*(-dtran*dx+xi1/m*(sin(psi)*sin(phi)+cos(psi)*cos(phi)*sin(theta)))+xi1/m*(sin(psi)*cos(phi)-cos(psi)*sin(phi)*sin(theta))*(p+sin(phi)*tan(theta)*q+cos(phi)*tan(theta)*r)+xi1/m*cos(psi)*cos(phi)*cos(theta)*(cos(phi)*q-sin(phi)*r)+xi1/m*(-cos(phi)*sin(psi)*sin(theta)+cos(psi)*sin(phi))*(sin(phi)/cos(theta)*q+cos(phi)/cos(theta)*r)+1/m*(sin(psi)*sin(phi)+cos(psi)*cos(phi)*sin(theta))*dxi1;
% % % output(5,1) = y;
% % % output(6,1) = dy;
% % % output(7,1) = -dtran*dy+xi1/m*(cos(phi)*sin(psi)*sin(theta)-cos(psi)*sin(phi));
% % % output(8,1) = -dtran*(-dtran*dy+xi1/m*(cos(phi)*sin(psi)*sin(theta)-cos(psi)*sin(phi)))+xi1/m*(-sin(phi)*sin(psi)*sin(theta)-cos(psi)*cos(phi))*(p+sin(phi)*tan(theta)*q+cos(phi)*tan(theta)*r)+xi1/m*sin(psi)*cos(phi)*cos(theta)*(cos(phi)*q-sin(phi)*r)+xi1/m*(sin(psi)*sin(phi)+cos(psi)*cos(phi)*sin(theta))*(sin(phi)/cos(theta)*q+cos(phi)/cos(theta)*r)+1/m*(cos(phi)*sin(psi)*sin(theta)-cos(psi)*sin(phi))*dxi1;
% % % output(9,1) = z;
% % % output(10,1) = dz;
% % % output(11,1) = -dtran*dz-m*g+xi1/m*cos(theta)*cos(phi);
% % % output(12,1) = -dtran*(-dtran*dz-m*g+xi1/m*cos(theta)*cos(phi))-xi1/m*cos(theta)*sin(phi)*(p+sin(phi)*tan(theta)*q+cos(phi)*tan(theta)*r)-xi1/m*sin(theta)*cos(phi)*(cos(phi)*q-sin(phi)*r)+1/m*cos(theta)*cos(phi)*dxi1 ;
% % % output(13,1) =  psi;
% % % output(14,1) = sin(phi)/cos(theta)*q+cos(phi)/cos(theta)*r;
% % %  
% % % 
% % % 
% % % xi = output;
